simulink model "MOD2_SMC"  (R2017a)
settings: Solver=FixedStepAuto  StartTime=0.0  StopTime=10  FixedStep=1/512000  RelTol=1e-3
libraries: dspmlti4 x4
settings Model: Creator=bhannigan  LastModifiedBy=bhannigan

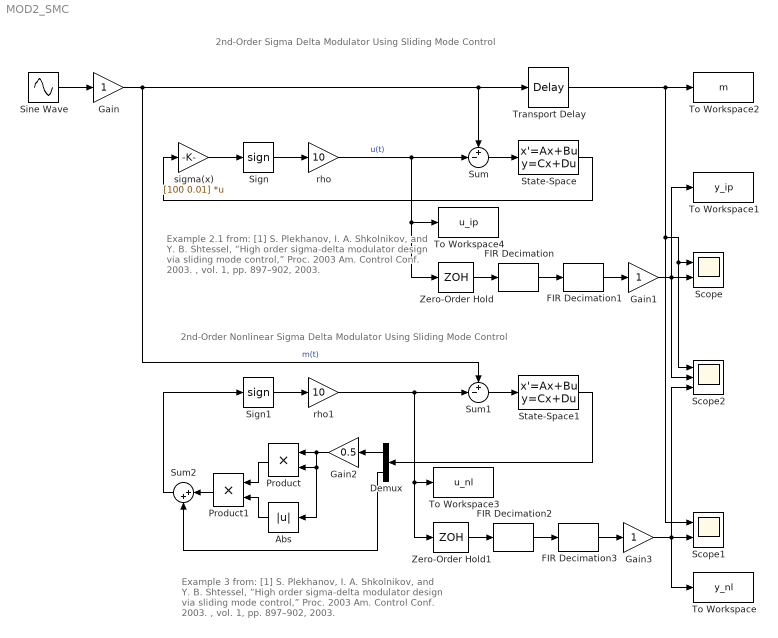
== system MOD2_SMC ==
  note: 2nd-Order Sigma Delta Modulator Using Sliding Mode Control
  note: Example 2.1 from:
      | [1] S. Plekhanov, I. A. Shkolnikov, and Y. B. Shtessel, “High order sigma-delta modulator design via sliding mode control,” Proc. 2003 Am. Control Conf. 2003. , vol. 1, pp. 897–902, 2003.
  note: 2nd-Order Nonlinear Sigma Delta Modulator Using Sliding Mode Control
  note: Example 3 from:
      | [1] S. Plekhanov, I. A. Shkolnikov, and Y. B. Shtessel, “High order sigma-delta modulator design via sliding mode control,” Proc. 2003 Am. Control Conf. 2003. , vol. 1, pp. 897–902, 2003.
  Abs : Abs
  Demux : Demux  Outputs=2
  FIR Decimation{,1..3} (4 alike) : dspmlti4/FIR Decimation  FilterSource=Dialog parameters  h=fir1(31,1/64)  D=8  filtStruct=Direct form  FilterObject=FDECIM  framing=Allow multirate processing  inputOffset=0  outputBufInitCond=0  roundingMode=Floor  overflowMode=off  firstCoeffDataTypeStr=Inherit: Same word length as input  firstCoeffMin=[]  firstCoeffMax=[]  firstCoeffLastDataTypeStr=Inherit: Same word length as input  outputDataTypeStr=Inherit: Same as accumulator  outputMin=[]  outputMax=[]  outputLastDataTypeStr=Inherit: Same as accumulator
  Gain : Gain
  Gain1 : Gain
  Gain2 : Gain  Gain=0.5
  Gain3 : Gain
  Product : Product
  Product1 : Product
  Scope : Scope  NumInputPorts=2
  Scope1 : Scope  NumInputPorts=2
  Scope2 : Scope  NumInputPorts=3
  Sign : Signum
  Sign1 : Signum
  Sine Wave : Sin  Frequency=2*pi*100  SampleTime=0
  State-Space : StateSpace  A=[0 1; 0 0]  B=[0; 1]  C=[1 0; 0 1]  D=[0; 0]  X0=0
  State-Space1 : StateSpace  A=[0 1; 0 0]  B=[0; 1]  C=[1 0; 0 1]  D=[0; 0]  X0=0
  Sum : Sum  Inputs=+-|
  Sum1 : Sum  Inputs=+-|
  Sum2 : Sum  Inputs=|++
  To Workspace : ToWorkspace  VariableName=y_nl  SaveFormat=Timeseries  SampleTime=-1
  To Workspace1 : ToWorkspace  VariableName=y_ip  SaveFormat=Timeseries  SampleTime=-1
  To Workspace2 : ToWorkspace  VariableName=m  SaveFormat=Timeseries  SampleTime=-1
  To Workspace3 : ToWorkspace  VariableName=u_nl  SaveFormat=Timeseries  SampleTime=-1
  To Workspace4 : ToWorkspace  VariableName=u_ip  SaveFormat=Timeseries  SampleTime=-1
  Transport Delay : TransportDelay  DelayTime=144/512000
  Zero-Order Hold : ZeroOrderHold  SampleTime=1/512000
  Zero-Order Hold1 : ZeroOrderHold  SampleTime=1/512000
  rho : Gain  Gain=10
  rho1 : Gain  Gain=10
  sigma(x) : Gain  Gain=[100 0.01]  Multiplication=Matrix(K*u) (u vector)
  wires:
  Sine Wave/1 -> Gain/1
  Gain/1 -> Sum1/1, Sum/1, Transport Delay/1  "m(t)"
  Sum/1 -> State-Space/1
  sigma(x)/1 -> Sign/1
  Sign/1 -> rho/1
  rho/1 -> To Workspace4/1, Zero-Order Hold/1, Sum/2  "u(t)"
  State-Space/1 -> sigma(x)/1
  FIR Decimation1/1 -> Gain1/1
  FIR Decimation/1 -> FIR Decimation1/1
  Zero-Order Hold/1 -> FIR Decimation/1
  Transport Delay/1 -> To Workspace2/1, Scope1/1, Scope2/1, Scope/1
  Sign1/1 -> rho1/1
  rho1/1 -> To Workspace3/1, Zero-Order Hold1/1, Sum1/2
  Sum1/1 -> State-Space1/1
  State-Space1/1 -> Demux/1
  Demux/1 -> Gain2/1
  Gain2/1 -> Abs/1, Product/2, Product/1
  Abs/1 -> Product1/2
  Product/1 -> Product1/1
  Product1/1 -> Sum2/1
  Demux/2 -> Sum2/2
  Sum2/1 -> Sign1/1
  FIR Decimation3/1 -> Gain3/1
  FIR Decimation2/1 -> FIR Decimation3/1
  Zero-Order Hold1/1 -> FIR Decimation2/1
  Gain3/1 -> To Workspace/1, Scope1/2, Scope2/3
  Gain1/1 -> To Workspace1/1, Scope/2, Scope2/2
